simulink model "model2bf"  (R2024b)
settings: Solver=ode4  StartTime=0.0  StopTime=20  FixedStep=2e-3  MaxStep=1e-1  RelTol=1e-3
values from neighbouring files (symbols this model uses):
  Aero = struct    [model2_dim.m]
  brake = struct    [model2_dim.m]
  drivetrain = struct    [model2_dim.m]
  g = 9.81    [model2_dim.m]
  G29 = struct    [model2_dim.m]
  hub_offset = 2.5    [model2_dim.m]
  motor = struct    [model2_dim.m]
  slope_angle = 0    [model2_dim.m]
  suspension = struct    [model2_dim.m]
  tyre = struct    [model2_dim.m]
  vehicle = struct    [model2_dim.m]
  Y = [vehicle.mt * 9.81; 0]    [braking_dyn.m]
undefined symbols (not defined in the file or in its folder): table, wheel, X, Z
libraries: sm_lib x154, nesl_utility x46, simulink x8, slrealtimeG29lib x1, Contact_Forces_Lib x1
(part 5 of 6)

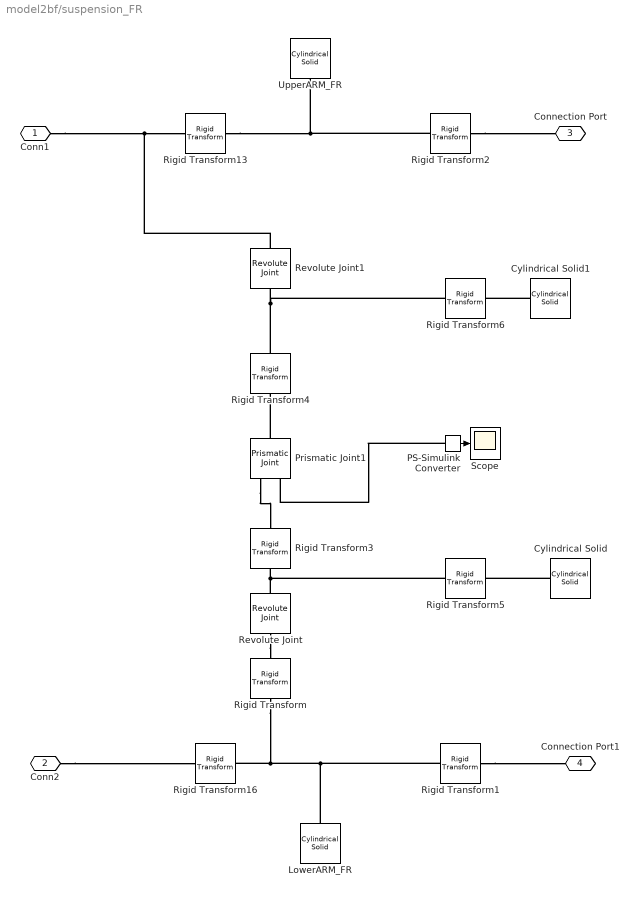
== system model2bf/suspension_FR ==
  Cylindrical Solid : sm_lib/Body Elements/Cylindrical Solid  CylinderRadius=1.5  CylinderRadiusUnits=cm  CylinderLength=15  CylinderLengthUnits=cm  ExportEntireGeometry=off  InertiaType=CalculateFromGeometry  BasedOnType=Density  Density=1000  DensityUnits=kg/m^3  Mass=1  MassUnits=kg  CenterOfMass=[0 0 0]  CenterOfMassUnits=m  MomentsOfInertia=[1 1 1]  MomentsOfInertiaUnits=kg*m^2  ProductsOfInertia=[0 0 0]  ProductsOfInertiaUnits=kg*m^2  GraphicType=FromGeometry  MarkerShape=Sphere  MarkerSize=10  GraphicVisPropType=SimpleVisualProperties  GraphicDiffuseColor=[0 0 1]  GraphicOpacity=1  GraphicSpecularColor=[0.5 0.5 0.5 1.0]  GraphicAmbientColor=[0.15 0.15 0.15 1.0]  GraphicEmissiveColor=[0.0 0.0 0.0 1.0]  GraphicShininess=75  DoExposeReferenceFrame=on  SerializedFrames=<Frames/>
  Cylindrical Solid1 : sm_lib/Body Elements/Cylindrical Solid  CylinderRadius=1  CylinderRadiusUnits=cm  CylinderLength=15  CylinderLengthUnits=cm  ExportEntireGeometry=off  InertiaType=CalculateFromGeometry  BasedOnType=Density  Density=1000  DensityUnits=kg/m^3  Mass=1  MassUnits=kg  CenterOfMass=[0 0 0]  CenterOfMassUnits=m  MomentsOfInertia=[1 1 1]  MomentsOfInertiaUnits=kg*m^2  ProductsOfInertia=[0 0 0]  ProductsOfInertiaUnits=kg*m^2  GraphicType=FromGeometry  MarkerShape=Sphere  MarkerSize=10  GraphicVisPropType=SimpleVisualProperties  GraphicDiffuseColor=[0.07451 0.6235 1]  GraphicOpacity=1  GraphicSpecularColor=[0.5 0.5 0.5 1.0]  GraphicAmbientColor=[0.15 0.15 0.15 1.0]  GraphicEmissiveColor=[0.0 0.0 0.0 1.0]  GraphicShininess=75  DoExposeReferenceFrame=on  SerializedFrames=<Frames/>
  LowerARM_FR : sm_lib/Body Elements/Cylindrical Solid  CylinderRadius=suspension.front.lower.radius  CylinderRadiusUnits=cm  CylinderLength=suspension.front.lower.length  CylinderLengthUnits=cm  ExportEntireGeometry=off  InertiaType=CalculateFromGeometry  BasedOnType=Density  Density=2700  DensityUnits=kg/m^3  Mass=1  MassUnits=kg  CenterOfMass=[0 0 0]  CenterOfMassUnits=m  MomentsOfInertia=[1 1 1]  MomentsOfInertiaUnits=kg*m^2  ProductsOfInertia=[0 0 0]  ProductsOfInertiaUnits=kg*m^2  GraphicType=FromGeometry  MarkerShape=Sphere  MarkerSize=10  GraphicVisPropType=SimpleVisualProperties  GraphicDiffuseColor=[0.5 0.5 0.5]  GraphicOpacity=1  GraphicSpecularColor=[0.5 0.5 0.5 1.0]  GraphicAmbientColor=[0.15 0.15 0.15 1.0]  GraphicEmissiveColor=[0.0 0.0 0.0 1.0]  GraphicShininess=75  DoExposeReferenceFrame=on  SerializedFrames=<Frames/>
  PS-Simulink Converter : nesl_utility/PS-Simulink Converter  PhysicalDomain=network_engine_domain  SubClassName=ps_output  LeftPortType=input  RightPortType=output  PseudoPeriodic=off  Frequencies=[]  VectorFormat=inherit  Unit=inherit  AffineConversion=off
  Prismatic Joint1 : sm_lib/Joints/Prismatic Joint  JointMode=Normal  CompositeWrenchDir=FollowerOnBase  CompositeWrenchFrame=BaseFrame  SenseConstraintForce=off  SenseConstraintTorque=off  SenseTotalForce=off  SenseTotalTorque=off  PositionTargetSpecify=off  PositionTargetPriority=High  PositionTargetValue=0  PositionTargetValueUnits=m  VelocityTargetSpecify=off  VelocityTargetPriority=High  VelocityTargetValue=0  VelocityTargetValueUnits=m/s  EquilibriumPosition=suspension.front.eq  EquilibriumPositionUnits=m  SpringStiffness=suspension.front.stiffness  SpringStiffnessUnits=N/m  DampingCoefficient=suspension.front.damping  DampingCoefficientUnits=N/(m/s)  LowerLimitSpecify=off  LowerLimitBound=-1  LowerLimitBoundUnits=m  LowerLimitStiffness=1e6  LowerLimitStiffnessUnits=N/m  LowerLimitDamping=1e3  LowerLimitDampingUnits=N/(m/s)  LowerLimitTransitionRegionWidth=1e-4  LowerLimitTransitionRegionWidthUnits=m  UpperLimitSpecify=off  UpperLimitBound=1  UpperLimitBoundUnits=m  UpperLimitStiffness=1e6  UpperLimitStiffnessUnits=N/m  UpperLimitDamping=1e3  UpperLimitDampingUnits=N/(m/s)  UpperLimitTransitionRegionWidth=1e-4  UpperLimitTransitionRegionWidthUnits=m  TorqueActuationMode=NoTorque  MotionActuationMode=ComputedMotion  SensePosition=on  SenseVelocity=off  SenseAcceleration=off  SenseTorqueForce=off  SenseLowerLimitTorqueForce=off  SenseUpperLimitTorqueForce=off
  Revolute Joint : sm_lib/Joints/Revolute Joint  JointMode=Normal  CompositeWrenchDir=FollowerOnBase  CompositeWrenchFrame=BaseFrame  SenseConstraintForce=off  SenseConstraintTorque=off  SenseTotalForce=off  SenseTotalTorque=off  PositionTargetSpecify=off  PositionTargetPriority=High  PositionTargetValue=0  PositionTargetValueUnits=deg  VelocityTargetSpecify=off  VelocityTargetPriority=High  VelocityTargetValue=0  VelocityTargetValueUnits=deg/s  EquilibriumPosition=0  EquilibriumPositionUnits=deg  SpringStiffness=0  SpringStiffnessUnits=N*m/deg  DampingCoefficient=0  DampingCoefficientUnits=N*m/(deg/s)  LowerLimitSpecify=off  LowerLimitBound=-90  LowerLimitBoundUnits=deg  LowerLimitStiffness=1e4  LowerLimitStiffnessUnits=N*m/deg  LowerLimitDamping=10  LowerLimitDampingUnits=N*m/(deg/s)  LowerLimitTransitionRegionWidth=0.1  LowerLimitTransitionRegionWidthUnits=deg  UpperLimitSpecify=off  UpperLimitBound=90  UpperLimitBoundUnits=deg  UpperLimitStiffness=1e4  UpperLimitStiffnessUnits=N*m/deg  UpperLimitDamping=10  UpperLimitDampingUnits=N*m/(deg/s)  UpperLimitTransitionRegionWidth=0.1  UpperLimitTransitionRegionWidthUnits=deg  TorqueActuationMode=NoTorque  MotionActuationMode=ComputedMotion  SensePosition=off  SenseVelocity=off  SenseAcceleration=off  SenseTorqueForce=off  SenseLowerLimitTorqueForce=off  SenseUpperLimitTorqueForce=off
  Revolute Joint1 : sm_lib/Joints/Revolute Joint  JointMode=Normal  CompositeWrenchDir=FollowerOnBase  CompositeWrenchFrame=BaseFrame  SenseConstraintForce=off  SenseConstraintTorque=off  SenseTotalForce=off  SenseTotalTorque=off  PositionTargetSpecify=off  PositionTargetPriority=High  PositionTargetValue=0  PositionTargetValueUnits=deg  VelocityTargetSpecify=off  VelocityTargetPriority=High  VelocityTargetValue=0  VelocityTargetValueUnits=deg/s  EquilibriumPosition=0  EquilibriumPositionUnits=deg  SpringStiffness=0  SpringStiffnessUnits=N*m/deg  DampingCoefficient=0  DampingCoefficientUnits=N*m/(deg/s)  LowerLimitSpecify=off  LowerLimitBound=-90  LowerLimitBoundUnits=deg  LowerLimitStiffness=1e4  LowerLimitStiffnessUnits=N*m/deg  LowerLimitDamping=10  LowerLimitDampingUnits=N*m/(deg/s)  LowerLimitTransitionRegionWidth=0.1  LowerLimitTransitionRegionWidthUnits=deg  UpperLimitSpecify=off  UpperLimitBound=90  UpperLimitBoundUnits=deg  UpperLimitStiffness=1e4  UpperLimitStiffnessUnits=N*m/deg  UpperLimitDamping=10  UpperLimitDampingUnits=N*m/(deg/s)  UpperLimitTransitionRegionWidth=0.1  UpperLimitTransitionRegionWidthUnits=deg  TorqueActuationMode=NoTorque  MotionActuationMode=ComputedMotion  SensePosition=off  SenseVelocity=off  SenseAcceleration=off  SenseTorqueForce=off  SenseLowerLimitTorqueForce=off  SenseUpperLimitTorqueForce=off
  Rigid Transform : sm_lib/Frames and Transforms/Rigid Transform  RotationMethod=StandardAxis  FollAlignAxisA=+X  BaseAlignAxisA=+Y  FollAlignAxisB=+Y  BaseAlignAxisB=+Z  RotationStandardAxis=+X  RotationAngle=-90  RotationAngleUnits=deg  RotationArbitraryAxis=[0 0 1]  RotationSequenceAxes=FollowerAxes  RotationSequence=XYX  RotationSequenceAngles=[0 0 0]  RotationSequenceAnglesUnits=deg  RotationMatrix=[1 0 0;0 1 0;0 0 1]  Quaternion=[1 0 0 0]  TranslationMethod=Cartesian  TranslationCartesianOffset=[0 0 -suspension.front.distance_revolute]  TranslationCartesianOffsetUnits=cm  TranslationStandardAxis=+Z  TranslationStandardOffset=0  TranslationStandardOffsetUnits=m  TranslationROffset=0  TranslationROffsetUnits=m  TranslationThetaOffset=0  TranslationThetaOffsetUnits=deg  TranslationZOffset=0  TranslationZOffsetUnits=m
  Rigid Transform1 : sm_lib/Frames and Transforms/Rigid Transform  RotationMethod=RotationSequence  FollAlignAxisA=+X  BaseAlignAxisA=+Y  FollAlignAxisB=+Y  BaseAlignAxisB=+Z  RotationStandardAxis=+X  RotationAngle=90  RotationAngleUnits=deg  RotationArbitraryAxis=[0 0 1]  RotationSequenceAxes=FollowerAxes  RotationSequence=XZX  RotationSequenceAngles=[90 suspension.front.lower.inclination 0]  RotationSequenceAnglesUnits=deg  RotationMatrix=[1 0 0;0 1 0;0 0 1]  Quaternion=[1 0 0 0]  TranslationMethod=Cartesian  TranslationCartesianOffset=[0 0 suspension.front.lower.length/2]  TranslationCartesianOffsetUnits=cm  TranslationStandardAxis=+Z  TranslationStandardOffset=0  TranslationStandardOffsetUnits=m  TranslationROffset=0  TranslationROffsetUnits=m  TranslationThetaOffset=0  TranslationThetaOffsetUnits=deg  TranslationZOffset=0  TranslationZOffsetUnits=m
  Rigid Transform13 : sm_lib/Frames and Transforms/Rigid Transform  RotationMethod=StandardAxis  FollAlignAxisA=+X  BaseAlignAxisA=+Y  FollAlignAxisB=+Y  BaseAlignAxisB=+Z  RotationStandardAxis=+X  RotationAngle=90  RotationAngleUnits=deg  RotationArbitraryAxis=[0 0 1]  RotationSequenceAxes=FollowerAxes  RotationSequence=XYX  RotationSequenceAngles=[0 0 0]  RotationSequenceAnglesUnits=deg  RotationMatrix=[1 0 0;0 1 0;0 0 1]  Quaternion=[1 0 0 0]  TranslationMethod=Cartesian  TranslationCartesianOffset=[0 -suspension.front.upper.length/2 0]  TranslationCartesianOffsetUnits=cm  TranslationStandardAxis=+Z  TranslationStandardOffset=0  TranslationStandardOffsetUnits=m  TranslationROffset=0  TranslationROffsetUnits=m  TranslationThetaOffset=0  TranslationThetaOffsetUnits=deg  TranslationZOffset=0  TranslationZOffsetUnits=m
  Rigid Transform16 : sm_lib/Frames and Transforms/Rigid Transform  RotationMethod=StandardAxis  FollAlignAxisA=+X  BaseAlignAxisA=+Y  FollAlignAxisB=+Y  BaseAlignAxisB=+Z  RotationStandardAxis=+X  RotationAngle=90  RotationAngleUnits=deg  RotationArbitraryAxis=[0 0 1]  RotationSequenceAxes=FollowerAxes  RotationSequence=XYX  RotationSequenceAngles=[0 0 0]  RotationSequenceAnglesUnits=deg  RotationMatrix=[1 0 0;0 1 0;0 0 1]  Quaternion=[1 0 0 0]  TranslationMethod=Cartesian  TranslationCartesianOffset=[0 -suspension.front.lower.length/2 0]  TranslationCartesianOffsetUnits=cm  TranslationStandardAxis=+Z  TranslationStandardOffset=0  TranslationStandardOffsetUnits=m  TranslationROffset=0  TranslationROffsetUnits=m  TranslationThetaOffset=0  TranslationThetaOffsetUnits=deg  TranslationZOffset=0  TranslationZOffsetUnits=m
  Rigid Transform2 : sm_lib/Frames and Transforms/Rigid Transform  RotationMethod=RotationSequence  FollAlignAxisA=+X  BaseAlignAxisA=+Y  FollAlignAxisB=+Y  BaseAlignAxisB=+Z  RotationStandardAxis=+X  RotationAngle=90  RotationAngleUnits=deg  RotationArbitraryAxis=[0 0 1]  RotationSequenceAxes=FollowerAxes  RotationSequence=XZX  RotationSequenceAngles=[90 suspension.front.upper.inclination 0]  RotationSequenceAnglesUnits=deg  RotationMatrix=[1 0 0;0 1 0;0 0 1]  Quaternion=[1 0 0 0]  TranslationMethod=Cartesian  TranslationCartesianOffset=[0 0 suspension.front.upper.length/2]  TranslationCartesianOffsetUnits=cm  TranslationStandardAxis=+Z  TranslationStandardOffset=0  TranslationStandardOffsetUnits=m  TranslationROffset=0  TranslationROffsetUnits=m  TranslationThetaOffset=0  TranslationThetaOffsetUnits=deg  TranslationZOffset=0  TranslationZOffsetUnits=m
  Rigid Transform3 : sm_lib/Frames and Transforms/Rigid Transform  RotationMethod=AlignedAxes  FollAlignAxisA=+Z  BaseAlignAxisA=-X  FollAlignAxisB=+Y  BaseAlignAxisB=+Z  RotationStandardAxis=+Y  RotationAngle=-90  RotationAngleUnits=deg  RotationArbitraryAxis=[0 0 1]  RotationSequenceAxes=FollowerAxes  RotationSequence=XYX  RotationSequenceAngles=[0 0 0]  RotationSequenceAnglesUnits=deg  RotationMatrix=[1 0 0;0 1 0;0 0 1]  Quaternion=[1 0 0 0]  TranslationMethod=None  TranslationCartesianOffset=[0 0 0]  TranslationCartesianOffsetUnits=m  TranslationStandardAxis=+Z  TranslationStandardOffset=0  TranslationStandardOffsetUnits=m  TranslationROffset=0  TranslationROffsetUnits=m  TranslationThetaOffset=0  TranslationThetaOffsetUnits=deg  TranslationZOffset=0  TranslationZOffsetUnits=m
  Rigid Transform4 : sm_lib/Frames and Transforms/Rigid Transform  RotationMethod=StandardAxis  FollAlignAxisA=+X  BaseAlignAxisA=+Y  FollAlignAxisB=+Y  BaseAlignAxisB=+Z  RotationStandardAxis=+X  RotationAngle=90  RotationAngleUnits=deg  RotationArbitraryAxis=[0 0 1]  RotationSequenceAxes=FollowerAxes  RotationSequence=XYX  RotationSequenceAngles=[0 0 0]  RotationSequenceAnglesUnits=deg  RotationMatrix=[1 0 0;0 1 0;0 0 1]  Quaternion=[1 0 0 0]  TranslationMethod=None  TranslationCartesianOffset=[0 0 0]  TranslationCartesianOffsetUnits=m  TranslationStandardAxis=+Z  TranslationStandardOffset=0  TranslationStandardOffsetUnits=m  TranslationROffset=0  TranslationROffsetUnits=m  TranslationThetaOffset=0  TranslationThetaOffsetUnits=deg  TranslationZOffset=0  TranslationZOffsetUnits=m
  Rigid Transform5 : sm_lib/Frames and Transforms/Rigid Transform  RotationMethod=StandardAxis  FollAlignAxisA=+X  BaseAlignAxisA=+Y  FollAlignAxisB=+Y  BaseAlignAxisB=+Z  RotationStandardAxis=+Y  RotationAngle=90  RotationAngleUnits=deg  RotationArbitraryAxis=[0 0 1]  RotationSequenceAxes=FollowerAxes  RotationSequence=XYX  RotationSequenceAngles=[0 0 0]  RotationSequenceAnglesUnits=deg  RotationMatrix=[1 0 0;0 1 0;0 0 1]  Quaternion=[1 0 0 0]  TranslationMethod=Cartesian  TranslationCartesianOffset=[0 0 7.5]  TranslationCartesianOffsetUnits=cm  TranslationStandardAxis=+Z  TranslationStandardOffset=0  TranslationStandardOffsetUnits=m  TranslationROffset=0  TranslationROffsetUnits=m  TranslationThetaOffset=0  TranslationThetaOffsetUnits=deg  TranslationZOffset=0  TranslationZOffsetUnits=m
  Rigid Transform6 : sm_lib/Frames and Transforms/Rigid Transform  RotationMethod=StandardAxis  FollAlignAxisA=+X  BaseAlignAxisA=+Y  FollAlignAxisB=+Y  BaseAlignAxisB=+Z  RotationStandardAxis=+X  RotationAngle=90  RotationAngleUnits=deg  RotationArbitraryAxis=[0 0 1]  RotationSequenceAxes=FollowerAxes  RotationSequence=XYX  RotationSequenceAngles=[0 0 0]  RotationSequenceAnglesUnits=deg  RotationMatrix=[1 0 0;0 1 0;0 0 1]  Quaternion=[1 0 0 0]  TranslationMethod=Cartesian  TranslationCartesianOffset=[0 0 7.5]  TranslationCartesianOffsetUnits=cm  TranslationStandardAxis=+Z  TranslationStandardOffset=0  TranslationStandardOffsetUnits=m  TranslationROffset=0  TranslationROffsetUnits=m  TranslationThetaOffset=0  TranslationThetaOffsetUnits=deg  TranslationZOffset=0  TranslationZOffsetUnits=m
  Scope : Scope
  UpperARM_FR : sm_lib/Body Elements/Cylindrical Solid  CylinderRadius=suspension.front.upper.radius  CylinderRadiusUnits=cm  CylinderLength=suspension.front.upper.length  CylinderLengthUnits=cm  ExportEntireGeometry=off  InertiaType=CalculateFromGeometry  BasedOnType=Density  Density=2700  DensityUnits=kg/m^3  Mass=1  MassUnits=kg  CenterOfMass=[0 0 0]  CenterOfMassUnits=m  MomentsOfInertia=[1 1 1]  MomentsOfInertiaUnits=kg*m^2  ProductsOfInertia=[0 0 0]  ProductsOfInertiaUnits=kg*m^2  GraphicType=FromGeometry  MarkerShape=Sphere  MarkerSize=10  GraphicVisPropType=SimpleVisualProperties  GraphicDiffuseColor=[1 0.4118 0.1608]  GraphicOpacity=1  GraphicSpecularColor=[0.5 0.5 0.5 1.0]  GraphicAmbientColor=[0.15 0.15 0.15 1.0]  GraphicEmissiveColor=[0.0 0.0 0.0 1.0]  GraphicShininess=75  DoExposeReferenceFrame=on  SerializedFrames=<Frames/>
  Conn1 : PMIOPort  Side=Left
  Conn2 : PMIOPort  Port=2  Side=Left
  Connection Port : PMIOPort  Port=3  Side=Right
  Connection Port1 : PMIOPort  Port=4  Side=Right
  wires:
  PS-Simulink Converter/1 -> Scope/1
  connections:
  Conn1/RConn1 -- Revolute Joint1/LConn1 -- Rigid Transform13/LConn1
  Conn2/RConn1 -- Rigid Transform16/LConn1
  LowerARM_FR/RConn1 -- Rigid Transform16/RConn1 -- Rigid Transform/LConn1 -- Rigid Transform1/LConn1
  Rigid Transform13/RConn1 -- Rigid Transform2/LConn1 -- UpperARM_FR/RConn1
  Rigid Transform1/RConn1 -- Connection Port1/RConn1
  Rigid Transform2/RConn1 -- Connection Port/RConn1
  Revolute Joint/LConn1 -- Rigid Transform5/RConn1 -- Rigid Transform3/LConn1
  Rigid Transform4/LConn1 -- Rigid Transform6/RConn1 -- Revolute Joint1/RConn1
  Cylindrical Solid1/RConn1 -- Rigid Transform6/LConn1
  Prismatic Joint1/LConn1 -- Rigid Transform4/RConn1
  Revolute Joint/RConn1 -- Rigid Transform/RConn1
  Cylindrical Solid/RConn1 -- Rigid Transform5/LConn1
  Prismatic Joint1/RConn1 -- Rigid Transform3/RConn1
  PS-Simulink Converter/LConn1 -- Prismatic Joint1/RConn2

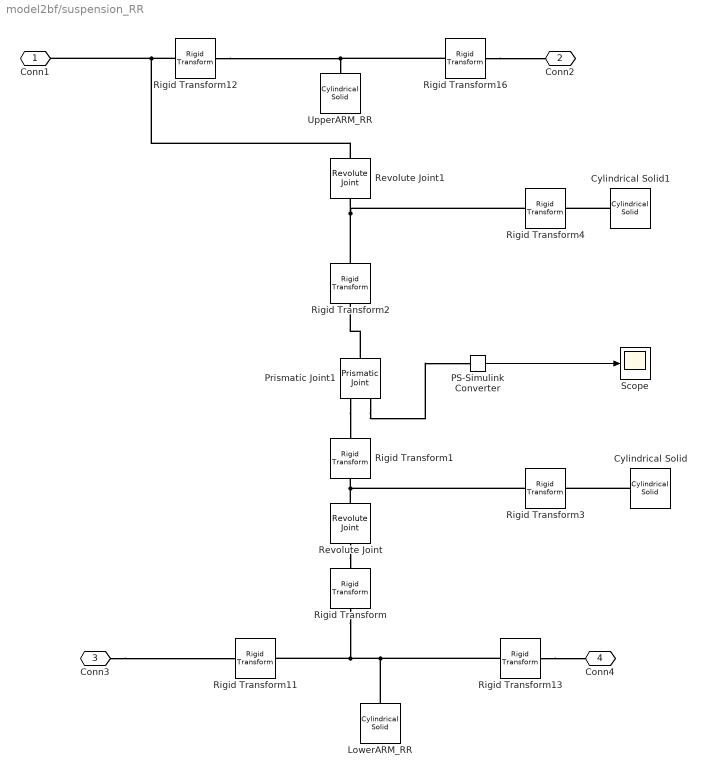
== system model2bf/suspension_RR ==
  Cylindrical Solid : sm_lib/Body Elements/Cylindrical Solid  CylinderRadius=1.5  CylinderRadiusUnits=cm  CylinderLength=15  CylinderLengthUnits=cm  ExportEntireGeometry=off  InertiaType=CalculateFromGeometry  BasedOnType=Density  Density=1000  DensityUnits=kg/m^3  Mass=1  MassUnits=kg  CenterOfMass=[0 0 0]  CenterOfMassUnits=m  MomentsOfInertia=[1 1 1]  MomentsOfInertiaUnits=kg*m^2  ProductsOfInertia=[0 0 0]  ProductsOfInertiaUnits=kg*m^2  GraphicType=FromGeometry  MarkerShape=Sphere  MarkerSize=10  GraphicVisPropType=SimpleVisualProperties  GraphicDiffuseColor=[0 0 1]  GraphicOpacity=1  GraphicSpecularColor=[0.5 0.5 0.5 1.0]  GraphicAmbientColor=[0.15 0.15 0.15 1.0]  GraphicEmissiveColor=[0.0 0.0 0.0 1.0]  GraphicShininess=75  DoExposeReferenceFrame=on  SerializedFrames=<Frames/>
  Cylindrical Solid1 : sm_lib/Body Elements/Cylindrical Solid  CylinderRadius=1  CylinderRadiusUnits=cm  CylinderLength=15  CylinderLengthUnits=cm  ExportEntireGeometry=off  InertiaType=CalculateFromGeometry  BasedOnType=Density  Density=1000  DensityUnits=kg/m^3  Mass=1  MassUnits=kg  CenterOfMass=[0 0 0]  CenterOfMassUnits=m  MomentsOfInertia=[1 1 1]  MomentsOfInertiaUnits=kg*m^2  ProductsOfInertia=[0 0 0]  ProductsOfInertiaUnits=kg*m^2  GraphicType=FromGeometry  MarkerShape=Sphere  MarkerSize=10  GraphicVisPropType=SimpleVisualProperties  GraphicDiffuseColor=[0.07451 0.6235 1]  GraphicOpacity=1  GraphicSpecularColor=[0.5 0.5 0.5 1.0]  GraphicAmbientColor=[0.15 0.15 0.15 1.0]  GraphicEmissiveColor=[0.0 0.0 0.0 1.0]  GraphicShininess=75  DoExposeReferenceFrame=on  SerializedFrames=<Frames/>
  LowerARM_RR : sm_lib/Body Elements/Cylindrical Solid  CylinderRadius=suspension.rear.lower.radius  CylinderRadiusUnits=cm  CylinderLength=suspension.rear.lower.length  CylinderLengthUnits=cm  ExportEntireGeometry=off  InertiaType=CalculateFromGeometry  BasedOnType=Density  Density=2700  DensityUnits=kg/m^3  Mass=1  MassUnits=kg  CenterOfMass=[0 0 0]  CenterOfMassUnits=m  MomentsOfInertia=[1 1 1]  MomentsOfInertiaUnits=kg*m^2  ProductsOfInertia=[0 0 0]  ProductsOfInertiaUnits=kg*m^2  GraphicType=FromGeometry  MarkerShape=Sphere  MarkerSize=10  GraphicVisPropType=SimpleVisualProperties  GraphicDiffuseColor=[0.5 0.5 0.5]  GraphicOpacity=1  GraphicSpecularColor=[0.5 0.5 0.5 1.0]  GraphicAmbientColor=[0.15 0.15 0.15 1.0]  GraphicEmissiveColor=[0.0 0.0 0.0 1.0]  GraphicShininess=75  DoExposeReferenceFrame=on  SerializedFrames=<Frames/>
  PS-Simulink Converter : nesl_utility/PS-Simulink Converter  PhysicalDomain=network_engine_domain  SubClassName=ps_output  LeftPortType=input  RightPortType=output  PseudoPeriodic=off  Frequencies=[]  VectorFormat=inherit  Unit=inherit  AffineConversion=off
  Prismatic Joint1 : sm_lib/Joints/Prismatic Joint  JointMode=Normal  CompositeWrenchDir=FollowerOnBase  CompositeWrenchFrame=BaseFrame  SenseConstraintForce=off  SenseConstraintTorque=off  SenseTotalForce=off  SenseTotalTorque=off  PositionTargetSpecify=off  PositionTargetPriority=High  PositionTargetValue=0  PositionTargetValueUnits=m  VelocityTargetSpecify=off  VelocityTargetPriority=High  VelocityTargetValue=0  VelocityTargetValueUnits=m/s  EquilibriumPosition=suspension.rear.eq  EquilibriumPositionUnits=m  SpringStiffness=suspension.rear.stiffness  SpringStiffnessUnits=N/m  DampingCoefficient=suspension.rear.damping  DampingCoefficientUnits=N/(m/s)  LowerLimitSpecify=off  LowerLimitBound=-1  LowerLimitBoundUnits=m  LowerLimitStiffness=1e6  LowerLimitStiffnessUnits=N/m  LowerLimitDamping=1e3  LowerLimitDampingUnits=N/(m/s)  LowerLimitTransitionRegionWidth=1e-4  LowerLimitTransitionRegionWidthUnits=m  UpperLimitSpecify=off  UpperLimitBound=1  UpperLimitBoundUnits=m  UpperLimitStiffness=1e6  UpperLimitStiffnessUnits=N/m  UpperLimitDamping=1e3  UpperLimitDampingUnits=N/(m/s)  UpperLimitTransitionRegionWidth=1e-4  UpperLimitTransitionRegionWidthUnits=m  TorqueActuationMode=NoTorque  MotionActuationMode=ComputedMotion  SensePosition=on  SenseVelocity=off  SenseAcceleration=off  SenseTorqueForce=off  SenseLowerLimitTorqueForce=off  SenseUpperLimitTorqueForce=off
  Revolute Joint : sm_lib/Joints/Revolute Joint  JointMode=Normal  CompositeWrenchDir=FollowerOnBase  CompositeWrenchFrame=BaseFrame  SenseConstraintForce=off  SenseConstraintTorque=off  SenseTotalForce=off  SenseTotalTorque=off  PositionTargetSpecify=off  PositionTargetPriority=High  PositionTargetValue=0  PositionTargetValueUnits=deg  VelocityTargetSpecify=off  VelocityTargetPriority=High  VelocityTargetValue=0  VelocityTargetValueUnits=deg/s  EquilibriumPosition=0  EquilibriumPositionUnits=deg  SpringStiffness=0  SpringStiffnessUnits=N*m/deg  DampingCoefficient=0  DampingCoefficientUnits=N*m/(deg/s)  LowerLimitSpecify=off  LowerLimitBound=-90  LowerLimitBoundUnits=deg  LowerLimitStiffness=1e4  LowerLimitStiffnessUnits=N*m/deg  LowerLimitDamping=10  LowerLimitDampingUnits=N*m/(deg/s)  LowerLimitTransitionRegionWidth=0.1  LowerLimitTransitionRegionWidthUnits=deg  UpperLimitSpecify=off  UpperLimitBound=90  UpperLimitBoundUnits=deg  UpperLimitStiffness=1e4  UpperLimitStiffnessUnits=N*m/deg  UpperLimitDamping=10  UpperLimitDampingUnits=N*m/(deg/s)  UpperLimitTransitionRegionWidth=0.1  UpperLimitTransitionRegionWidthUnits=deg  TorqueActuationMode=NoTorque  MotionActuationMode=ComputedMotion  SensePosition=off  SenseVelocity=off  SenseAcceleration=off  SenseTorqueForce=off  SenseLowerLimitTorqueForce=off  SenseUpperLimitTorqueForce=off
  Revolute Joint1 : sm_lib/Joints/Revolute Joint  JointMode=Normal  CompositeWrenchDir=FollowerOnBase  CompositeWrenchFrame=BaseFrame  SenseConstraintForce=off  SenseConstraintTorque=off  SenseTotalForce=off  SenseTotalTorque=off  PositionTargetSpecify=off  PositionTargetPriority=High  PositionTargetValue=0  PositionTargetValueUnits=deg  VelocityTargetSpecify=off  VelocityTargetPriority=High  VelocityTargetValue=0  VelocityTargetValueUnits=deg/s  EquilibriumPosition=0  EquilibriumPositionUnits=deg  SpringStiffness=0  SpringStiffnessUnits=N*m/deg  DampingCoefficient=0  DampingCoefficientUnits=N*m/(deg/s)  LowerLimitSpecify=off  LowerLimitBound=-90  LowerLimitBoundUnits=deg  LowerLimitStiffness=1e4  LowerLimitStiffnessUnits=N*m/deg  LowerLimitDamping=10  LowerLimitDampingUnits=N*m/(deg/s)  LowerLimitTransitionRegionWidth=0.1  LowerLimitTransitionRegionWidthUnits=deg  UpperLimitSpecify=off  UpperLimitBound=90  UpperLimitBoundUnits=deg  UpperLimitStiffness=1e4  UpperLimitStiffnessUnits=N*m/deg  UpperLimitDamping=10  UpperLimitDampingUnits=N*m/(deg/s)  UpperLimitTransitionRegionWidth=0.1  UpperLimitTransitionRegionWidthUnits=deg  TorqueActuationMode=NoTorque  MotionActuationMode=ComputedMotion  SensePosition=off  SenseVelocity=off  SenseAcceleration=off  SenseTorqueForce=off  SenseLowerLimitTorqueForce=off  SenseUpperLimitTorqueForce=off
  Rigid Transform : sm_lib/Frames and Transforms/Rigid Transform  RotationMethod=StandardAxis  FollAlignAxisA=+X  BaseAlignAxisA=+Y  FollAlignAxisB=+Y  BaseAlignAxisB=+Z  RotationStandardAxis=+X  RotationAngle=-90  RotationAngleUnits=deg  RotationArbitraryAxis=[0 0 1]  RotationSequenceAxes=FollowerAxes  RotationSequence=XYX  RotationSequenceAngles=[0 0 0]  RotationSequenceAnglesUnits=deg  RotationMatrix=[1 0 0;0 1 0;0 0 1]  Quaternion=[1 0 0 0]  TranslationMethod=Cartesian  TranslationCartesianOffset=[0 0 -suspension.rear.distance_revolute]  TranslationCartesianOffsetUnits=cm  TranslationStandardAxis=+Z  TranslationStandardOffset=0  TranslationStandardOffsetUnits=m  TranslationROffset=0  TranslationROffsetUnits=m  TranslationThetaOffset=0  TranslationThetaOffsetUnits=deg  TranslationZOffset=0  TranslationZOffsetUnits=m
  Rigid Transform1 : sm_lib/Frames and Transforms/Rigid Transform  RotationMethod=AlignedAxes  FollAlignAxisA=+Z  BaseAlignAxisA=-X  FollAlignAxisB=+Y  BaseAlignAxisB=+Z  RotationStandardAxis=+Y  RotationAngle=-90  RotationAngleUnits=deg  RotationArbitraryAxis=[0 0 1]  RotationSequenceAxes=FollowerAxes  RotationSequence=XYX  RotationSequenceAngles=[0 0 0]  RotationSequenceAnglesUnits=deg  RotationMatrix=[1 0 0;0 1 0;0 0 1]  Quaternion=[1 0 0 0]  TranslationMethod=None  TranslationCartesianOffset=[0 0 0]  TranslationCartesianOffsetUnits=m  TranslationStandardAxis=+Z  TranslationStandardOffset=0  TranslationStandardOffsetUnits=m  TranslationROffset=0  TranslationROffsetUnits=m  TranslationThetaOffset=0  TranslationThetaOffsetUnits=deg  TranslationZOffset=0  TranslationZOffsetUnits=m
  Rigid Transform11 : sm_lib/Frames and Transforms/Rigid Transform  RotationMethod=StandardAxis  FollAlignAxisA=+X  BaseAlignAxisA=+Y  FollAlignAxisB=+Y  BaseAlignAxisB=+Z  RotationStandardAxis=+X  RotationAngle=90  RotationAngleUnits=deg  RotationArbitraryAxis=[0 0 1]  RotationSequenceAxes=FollowerAxes  RotationSequence=XYX  RotationSequenceAngles=[0 0 0]  RotationSequenceAnglesUnits=deg  RotationMatrix=[1 0 0;0 1 0;0 0 1]  Quaternion=[1 0 0 0]  TranslationMethod=Cartesian  TranslationCartesianOffset=[0 -suspension.rear.lower.length/2 0]  TranslationCartesianOffsetUnits=cm  TranslationStandardAxis=+Z  TranslationStandardOffset=0  TranslationStandardOffsetUnits=m  TranslationROffset=0  TranslationROffsetUnits=m  TranslationThetaOffset=0  TranslationThetaOffsetUnits=deg  TranslationZOffset=0  TranslationZOffsetUnits=m
  Rigid Transform12 : sm_lib/Frames and Transforms/Rigid Transform  RotationMethod=StandardAxis  FollAlignAxisA=+X  BaseAlignAxisA=+Y  FollAlignAxisB=+Y  BaseAlignAxisB=+Z  RotationStandardAxis=+X  RotationAngle=90  RotationAngleUnits=deg  RotationArbitraryAxis=[0 0 1]  RotationSequenceAxes=FollowerAxes  RotationSequence=XYX  RotationSequenceAngles=[0 0 0]  RotationSequenceAnglesUnits=deg  RotationMatrix=[1 0 0;0 1 0;0 0 1]  Quaternion=[1 0 0 0]  TranslationMethod=Cartesian  TranslationCartesianOffset=[0 -suspension.rear.upper.length/2 0]  TranslationCartesianOffsetUnits=cm  TranslationStandardAxis=+Z  TranslationStandardOffset=0  TranslationStandardOffsetUnits=m  TranslationROffset=0  TranslationROffsetUnits=m  TranslationThetaOffset=0  TranslationThetaOffsetUnits=deg  TranslationZOffset=0  TranslationZOffsetUnits=m
  Rigid Transform13 : sm_lib/Frames and Transforms/Rigid Transform  RotationMethod=RotationSequence  FollAlignAxisA=+X  BaseAlignAxisA=+Y  FollAlignAxisB=+Y  BaseAlignAxisB=+Z  RotationStandardAxis=+X  RotationAngle=90  RotationAngleUnits=deg  RotationArbitraryAxis=[0 0 1]  RotationSequenceAxes=FollowerAxes  RotationSequence=XZX  RotationSequenceAngles=[90 suspension.rear.lower.inclination 0]  RotationSequenceAnglesUnits=deg  RotationMatrix=[1 0 0;0 1 0;0 0 1]  Quaternion=[1 0 0 0]  TranslationMethod=Cartesian  TranslationCartesianOffset=[0 0 suspension.rear.lower.length/2]  TranslationCartesianOffsetUnits=cm  TranslationStandardAxis=+Z  TranslationStandardOffset=0  TranslationStandardOffsetUnits=m  TranslationROffset=0  TranslationROffsetUnits=m  TranslationThetaOffset=0  TranslationThetaOffsetUnits=deg  TranslationZOffset=0  TranslationZOffsetUnits=m
  Rigid Transform16 : sm_lib/Frames and Transforms/Rigid Transform  RotationMethod=RotationSequence  FollAlignAxisA=+X  BaseAlignAxisA=+Y  FollAlignAxisB=+Y  BaseAlignAxisB=+Z  RotationStandardAxis=+X  RotationAngle=90  RotationAngleUnits=deg  RotationArbitraryAxis=[0 0 1]  RotationSequenceAxes=FollowerAxes  RotationSequence=XZX  RotationSequenceAngles=[90 suspension.rear.upper.inclination 0]  RotationSequenceAnglesUnits=deg  RotationMatrix=[1 0 0;0 1 0;0 0 1]  Quaternion=[1 0 0 0]  TranslationMethod=Cartesian  TranslationCartesianOffset=[0 0 suspension.rear.upper.length/2]  TranslationCartesianOffsetUnits=cm  TranslationStandardAxis=+Z  TranslationStandardOffset=0  TranslationStandardOffsetUnits=m  TranslationROffset=0  TranslationROffsetUnits=m  TranslationThetaOffset=0  TranslationThetaOffsetUnits=deg  TranslationZOffset=0  TranslationZOffsetUnits=m
  Rigid Transform2 : sm_lib/Frames and Transforms/Rigid Transform  RotationMethod=StandardAxis  FollAlignAxisA=+X  BaseAlignAxisA=+Y  FollAlignAxisB=+Y  BaseAlignAxisB=+Z  RotationStandardAxis=+X  RotationAngle=90  RotationAngleUnits=deg  RotationArbitraryAxis=[0 0 1]  RotationSequenceAxes=FollowerAxes  RotationSequence=XYX  RotationSequenceAngles=[0 0 0]  RotationSequenceAnglesUnits=deg  RotationMatrix=[1 0 0;0 1 0;0 0 1]  Quaternion=[1 0 0 0]  TranslationMethod=None  TranslationCartesianOffset=[0 0 0]  TranslationCartesianOffsetUnits=m  TranslationStandardAxis=+Z  TranslationStandardOffset=0  TranslationStandardOffsetUnits=m  TranslationROffset=0  TranslationROffsetUnits=m  TranslationThetaOffset=0  TranslationThetaOffsetUnits=deg  TranslationZOffset=0  TranslationZOffsetUnits=m
  Rigid Transform3 : sm_lib/Frames and Transforms/Rigid Transform  RotationMethod=StandardAxis  FollAlignAxisA=+X  BaseAlignAxisA=+Y  FollAlignAxisB=+Y  BaseAlignAxisB=+Z  RotationStandardAxis=+Y  RotationAngle=90  RotationAngleUnits=deg  RotationArbitraryAxis=[0 0 1]  RotationSequenceAxes=FollowerAxes  RotationSequence=XYX  RotationSequenceAngles=[0 0 0]  RotationSequenceAnglesUnits=deg  RotationMatrix=[1 0 0;0 1 0;0 0 1]  Quaternion=[1 0 0 0]  TranslationMethod=Cartesian  TranslationCartesianOffset=[0 0 7.5]  TranslationCartesianOffsetUnits=cm  TranslationStandardAxis=+Z  TranslationStandardOffset=0  TranslationStandardOffsetUnits=m  TranslationROffset=0  TranslationROffsetUnits=m  TranslationThetaOffset=0  TranslationThetaOffsetUnits=deg  TranslationZOffset=0  TranslationZOffsetUnits=m
  Rigid Transform4 : sm_lib/Frames and Transforms/Rigid Transform  RotationMethod=StandardAxis  FollAlignAxisA=+X  BaseAlignAxisA=+Y  FollAlignAxisB=+Y  BaseAlignAxisB=+Z  RotationStandardAxis=+X  RotationAngle=90  RotationAngleUnits=deg  RotationArbitraryAxis=[0 0 1]  RotationSequenceAxes=FollowerAxes  RotationSequence=XYX  RotationSequenceAngles=[0 0 0]  RotationSequenceAnglesUnits=deg  RotationMatrix=[1 0 0;0 1 0;0 0 1]  Quaternion=[1 0 0 0]  TranslationMethod=Cartesian  TranslationCartesianOffset=[0 0 7.5]  TranslationCartesianOffsetUnits=cm  TranslationStandardAxis=+Z  TranslationStandardOffset=0  TranslationStandardOffsetUnits=m  TranslationROffset=0  TranslationROffsetUnits=m  TranslationThetaOffset=0  TranslationThetaOffsetUnits=deg  TranslationZOffset=0  TranslationZOffsetUnits=m
  Scope : Scope
  UpperARM_RR : sm_lib/Body Elements/Cylindrical Solid  CylinderRadius=suspension.rear.upper.radius  CylinderRadiusUnits=cm  CylinderLength=suspension.rear.upper.length  CylinderLengthUnits=cm  ExportEntireGeometry=off  InertiaType=CalculateFromGeometry  BasedOnType=Density  Density=2700  DensityUnits=kg/m^3  Mass=1  MassUnits=kg  CenterOfMass=[0 0 0]  CenterOfMassUnits=m  MomentsOfInertia=[1 1 1]  MomentsOfInertiaUnits=kg*m^2  ProductsOfInertia=[0 0 0]  ProductsOfInertiaUnits=kg*m^2  GraphicType=FromGeometry  MarkerShape=Sphere  MarkerSize=10  GraphicVisPropType=SimpleVisualProperties  GraphicDiffuseColor=[1 0.4118 0.1608]  GraphicOpacity=1  GraphicSpecularColor=[0.5 0.5 0.5 1.0]  GraphicAmbientColor=[0.15 0.15 0.15 1.0]  GraphicEmissiveColor=[0.0 0.0 0.0 1.0]  GraphicShininess=75  DoExposeReferenceFrame=on  SerializedFrames=<Frames/>
  Conn1 : PMIOPort  Side=Left
  Conn2 : PMIOPort  Port=2  Side=Right
  Conn3 : PMIOPort  Port=3  Side=Left
  Conn4 : PMIOPort  Port=4  Side=Right
  wires:
  PS-Simulink Converter/1 -> Scope/1
  connections:
  Rigid Transform13/RConn1 -- Conn4/RConn1
  Rigid Transform16/RConn1 -- Conn2/RConn1
  LowerARM_RR/RConn1 -- Rigid Transform13/LConn1 -- Rigid Transform/LConn1 -- Rigid Transform11/RConn1
  Rigid Transform12/RConn1 -- Rigid Transform16/LConn1 -- UpperARM_RR/RConn1
  Rigid Transform12/LConn1 -- Conn1/RConn1 -- Revolute Joint1/LConn1
  Conn3/RConn1 -- Rigid Transform11/LConn1
  Revolute Joint/RConn1 -- Rigid Transform/RConn1
  Revolute Joint/LConn1 -- Rigid Transform3/RConn1 -- Rigid Transform1/LConn1
  Rigid Transform2/LConn1 -- Rigid Transform4/RConn1 -- Revolute Joint1/RConn1
  Prismatic Joint1/LConn1 -- Rigid Transform2/RConn1
  Cylindrical Solid/RConn1 -- Rigid Transform3/LConn1
  Cylindrical Solid1/RConn1 -- Rigid Transform4/LConn1
  Prismatic Joint1/RConn1 -- Rigid Transform1/RConn1
  Prismatic Joint1/RConn2 -- PS-Simulink Converter/LConn1

== system model2bf/Chassis/Aero Forces ==
  u : Inport
  Constant : Constant
  Constant1 : Constant  Value=0
  Gain : Gain  Gain=[-Aero.Drag_reduced, 0, Aero.Lift_reduced]
  MATLAB Function : MATLAB Function  TreatAsAtomicUnit=on
  Product : Product
  Switch : Switch  Criteria=u2 > Threshold  SaturateOnIntegerOverflow=off  InputSameDT=off
  Out1 : Outport
  wires:
  MATLAB Function/1(y) -> Switch/2, Product/2
  Constant1/1 -> Switch/3
  Gain/1 -> Out1/1
  Constant/1 -> Switch/1
  Switch/1 -> Product/1
  Product/1 -> Gain/1
  u/1 -> MATLAB Function/1(u)

== system model2bf/Driveline/Acceleration calculation ==
  wheel force : Inport
  Abs : Abs  SaturateOnIntegerOverflow=off
  From : From  Commented=on  GotoTag=Fy_RL  TagVisibility=global
  From1 : From  Commented=on  GotoTag=Fy_RR  TagVisibility=global
  Gain : Gain  Commented=on  Gain=motor.efficiency*motor.gearratio/(tyre.radius/100)
  Gain1 : Gain  Gain=1/((wheel.ir1+wheel.ir2+drivetrain.i_tot*motor.gearratio^2)/((tyre.radius/100)*(tyre.dynamic_radius/100))+vehicle.totalmass)
  MATLAB Function : MATLAB Function  Commented=on  TreatAsAtomicUnit=on
  Min : MinMax  Commented=on  Inputs=2
  Minus : Sum  Inputs=+---
  Rolling coefficient term : Constant  Value=tyre.Cr*vehicle.totalmass*g*cosd(slope_angle)
  Scope : Scope
  Scope1 : Scope
  Slope term : Constant  Value=vehicle.totalmass*g*sind(slope_angle)
  mu_a : Gain  Commented=on  Gain=vehicle.mu_a
  mu_g : Gain  Commented=on  Gain=vehicle.mu_g
  Acceleration : Outport
  wires:
  Rolling coefficient term/1 -> Minus/3
  Slope term/1 -> Minus/4
  Minus/1 -> Gain1/1
  Gain1/1 -> Scope1/1, Acceleration/1
  Min/1 -> mu_g/1, mu_a/1
  mu_a/1 -> MATLAB Function/1(maxforce)
  mu_g/1 -> MATLAB Function/2(limitforce)
  Gain/1 -> MATLAB Function/3(wheelforce)
  wheel force/1 -> Scope/1, Minus/1
  From/1 -> Min/1
  From1/1 -> Min/2
  Abs/1 -> Minus/2
  [F_D] -> Abs/1

== system model2bf/Driveline/Subsystem2 ==
  v (m/s) : Inport
  Braking (%) : Inport  Port=2
  Because we cannot use regen braking at low speed : Switch  Criteria=u2 > Threshold  Threshold=2  SaturateOnIntegerOverflow=off  InputSameDT=off
  Constant : Constant  Value=0
  Gain : Gain  Gain=1 - brake.brakefraction
  Gain1 : Gain  Gain=brake.brakefraction
  Gain2 : Gain  Gain=1/motor.gearratio
  Gain3 : Gain  Gain=brake.pedalratio
  Gain4 : Gain  Gain=1/brake.mastercylinderA
  Gain5 : Gain  Gain=brake.pistonN*brake.pistonA
  Gain6 : Gain  Gain=2*brake.effectiveradius*brake.padfriction
  Gain7 : Gain  Gain=brake.Ffoot_max
  Saturation : Saturate  UpperLimit=0  LowerLimit=-500
  Switch : Switch  Criteria=u2 > Threshold  Threshold=2  SaturateOnIntegerOverflow=off  InputSameDT=off
  FrictionBrake_Tr : Outport
  RegenBrake_Tr : Outport  Port=2
  wires:
  Gain1/1 -> Gain2/1  "RegenBrakeWheel_Tr"
  v (m/s)/1 -> Because we cannot use regen braking at low speed/2, Switch/2
  Constant/1 -> Because we cannot use regen braking at low speed/3
  Switch/1 -> FrictionBrake_Tr/1  "FrictionBrake_Tr"
  Saturation/1 -> RegenBrake_Tr/1  "RegenBrakeTrq"
  Because we cannot use regen braking at low speed/1 -> Saturation/1
  Gain/1 -> Switch/1  "FrictionBrake_Tr"
  Gain6/1 -> Switch/3, Gain1/1, Gain/1  "Total_brake_Tr"
  Gain5/1 -> Gain6/1  "F_clamp"
  Gain4/1 -> Gain5/1  "P_line"
  Gain3/1 -> Gain4/1  "F_pedal"
  Braking (%)/1 -> Gain7/1
  Gain7/1 -> Gain3/1  "F_foot"
  Gain2/1 -> Because we cannot use regen braking at low speed/1  "RegenBrakeMotor_Tr"

== system model2bf/Driveline/Subsystem3 ==
  Motor torque (Nm) : Inport
  Regen Torque : Inport  Port=2
  Throttle (%) : Inport  Port=3
  Add : Sum
  Subsystem : Subsystem
  Torque limit : Subsystem
  MotorTrqOut (Nm) : Outport
  wires:
  Regen Torque/1 -> Subsystem/1(Regen_demand)
  Torque limit/1(Regen_trq_limit) -> Subsystem/2(Regen_Limit)
  Subsystem/1(Regen_Trq) -> Add/1
  Throttle (%)/1 -> Torque limit/1(Throttle (%))
  Motor torque (Nm)/1 -> Torque limit/2(Motor torque (Nm))
  Torque limit/2(Trq_Dmd) -> Add/2
  Add/1 -> MotorTrqOut (Nm)/1  "mech. torque"

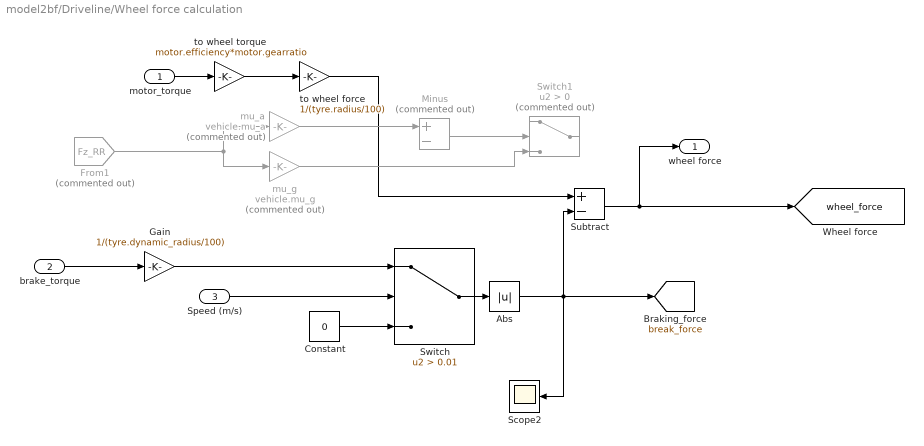
== system model2bf/Driveline/Wheel force calculation ==
  motor_torque : Inport
  brake_torque : Inport  Port=2
  Speed (m/s) : Inport  Port=3
  Abs : Abs  SaturateOnIntegerOverflow=off
  Constant : Constant  Value=0
  From1 : From  Commented=on  GotoTag=Fz_RR  TagVisibility=global
  Gain : Gain  Gain=1/(tyre.dynamic_radius/100)
  Minus : Sum  Commented=on  Inputs=+-
  Scope2 : Scope
  Subtract : Sum  Inputs=+-
  Switch : Switch  Criteria=u2 > Threshold  Threshold=0.01  SaturateOnIntegerOverflow=off  InputSameDT=off
  Switch1 : Switch  Commented=on  Criteria=u2 > Threshold  SaturateOnIntegerOverflow=off  InputSameDT=off
  mu_a : Gain  Commented=on  Gain=vehicle.mu_a
  mu_g : Gain  Commented=on  Gain=vehicle.mu_g
  to wheel force : Gain  Gain=1/(tyre.radius/100)
  to wheel torque : Gain  Gain=motor.efficiency*motor.gearratio
  wheel force : Outport
  tag scope: break_force=global, wheel_force=global
  wires:
  motor_torque/1 -> to wheel torque/1
  to wheel torque/1 -> to wheel force/1
  brake_torque/1 -> Gain/1
  Gain/1 -> Switch/1
  Speed (m/s)/1 -> Switch/2
  Constant/1 -> Switch/3
  Switch/1 -> Abs/1
  to wheel force/1 -> Subtract/1
  Subtract/1 -> wheel force/1, [wheel_force]
  Abs/1 -> Scope2/1, Subtract/2, [break_force]
  From1/1 -> mu_g/1, mu_a/1
  mu_g/1 -> Switch1/3
  mu_a/1 -> Minus/1
  Minus/1 -> Switch1/2

== system model2bf/Tyre FR/Magic formula subsystem ==
  note: SIgn of the steering input
  note: positive force = to the left
  Fz : Inport
  Steering input : Inport  Port=2
  Tyre data : Inport  Port=3
  Bus Selector : BusSelector  OutputSignals=velocity_FR,rotation_FR,inclination_FR
  Constant : Constant  Value=0
  MATLAB Function : MATLAB Function  TreatAsAtomicUnit=on
  Magic formula : MATLAB Function  TreatAsAtomicUnit=on
  Scope : Scope
  Scope1 : Scope
  Sum : Sum
  Switch : Switch  Criteria=u2 > Threshold  Threshold=0.5  SaturateOnIntegerOverflow=off  InputSameDT=off
  norm : MATLAB Function  TreatAsAtomicUnit=on
  Force : Outport
  wires:
  Fz/1 -> Magic formula/1(Fz)
  Switch/1 -> Force/1
  norm/1(y) -> Switch/2
  Magic formula/1(Fy) -> Scope/1, Switch/1
  Constant/1 -> Switch/3
  Tyre data/1 -> Bus Selector/1
  Steering input/1 -> Sum/1
  MATLAB Function/1(theta) -> Scope1/1, Sum/2  "slip angle"
  Sum/1 -> Magic formula/2(SA)  "Effective slip angle_FR"
  Bus Selector/1 -> [Speed], MATLAB Function/1(u)  "<velocity_FR>"
  [Speed] -> norm/1(u)
  Bus Selector/2 -> MATLAB Function/2(r)  "<rotation_FR>"
  Bus Selector/3 -> Magic formula/3(Camber)  "<inclination_FR>"

== system model2bf/Tyre_FL/Magic formula subsystem ==
  note: reflection
      | : positive slip = tyre turned to the left = force to the left
  note: SIgn of the steering input
  note: positive force = to the left
  Fz : Inport
  Steering input : Inport  Port=2
  Tyre data : Inport  Port=3
  Bus Selector : BusSelector  OutputSignals=velocity_FL,rotation_FL,inclination_FL
  Constant : Constant  Value=0
  MATLAB Function : MATLAB Function  TreatAsAtomicUnit=on
  Magic formula : MATLAB Function  TreatAsAtomicUnit=on
  Scope : Scope
  Scope1 : Scope
  Sum : Sum
  Switch : Switch  Criteria=u2 > Threshold  Threshold=0.5  SaturateOnIntegerOverflow=off  InputSameDT=off
  norm : MATLAB Function  TreatAsAtomicUnit=on
  Force : Outport
  wires:
  Fz/1 -> Magic formula/1(Fz)
  Switch/1 -> Force/1
  norm/1(y) -> Switch/2
  Magic formula/1(Fy) -> Scope/1, Switch/1
  Constant/1 -> Switch/3
  Tyre data/1 -> Bus Selector/1
  Steering input/1 -> Sum/1
  MATLAB Function/1(theta) -> Sum/2, Scope1/1  "slip angle"
  Sum/1 -> Magic formula/2(SA)  "Effective slip angle_FL"
  Bus Selector/1 -> MATLAB Function/1(u), [Speed]  "<velocity_FL>"
  [Speed] -> norm/1(u)
  Bus Selector/2 -> MATLAB Function/2(r)  "<rotation_FL>"
  Bus Selector/3 -> Magic formula/3(Camber)  "<inclination_FL>"

== system model2bf/Tyre_RL/Magic formula subsystem ==
  note: positive force = to the left
  Fz : Inport
  Tyre data : Inport  Port=2
  Bus Selector : BusSelector  OutputSignals=velocity_RL,rotation_RL,inclination_RL
  Constant : Constant  Value=0
  MATLAB Function : MATLAB Function  TreatAsAtomicUnit=on
  Magic formula : MATLAB Function  TreatAsAtomicUnit=on
  Scope : Scope
  Scope1 : Scope
  Switch : Switch  Criteria=u2 > Threshold  Threshold=0.5  SaturateOnIntegerOverflow=off  InputSameDT=off
  norm : MATLAB Function  TreatAsAtomicUnit=on
  Force : Outport
  wires:
  Fz/1 -> Magic formula/1(Fz)
  Switch/1 -> Force/1
  norm/1(y) -> Switch/2
  Magic formula/1(Fy) -> Scope/1, Switch/1
  Constant/1 -> Switch/3
  Tyre data/1 -> Bus Selector/1
  MATLAB Function/1(theta) -> Magic formula/2(SA), Scope1/1  "Effective slip angle_RL"
  Bus Selector/1 -> [Speed], MATLAB Function/1(u)  "<velocity_RL>"
  [Speed] -> norm/1(u)
  Bus Selector/2 -> MATLAB Function/2(r)  "<rotation_RL>"
  Bus Selector/3 -> Magic formula/3(Camber)  "<inclination_RL>"

== system model2bf/Tyre_RL/Subsystem ==
  Constant{,1..3} (4 alike) : Constant  Value=0
  Vector Concatenate : Concatenate  NumInputs=3
  Vector Concatenate1 : Concatenate  NumInputs=3
  Vector Concatenate3 : Concatenate  NumInputs=3
  inclination_RL : Outport
  inclination_RL1 : Outport  Port=2
  inclination_RL2 : Outport  Port=3
  inclination_RL3 : Outport  Port=4
  wires:
  Constant/1 -> Vector Concatenate/3, Vector Concatenate/2, Vector Concatenate/1
  Vector Concatenate/1 -> inclination_RL/1  "inclination_RL"
  Constant1/1 -> Vector Concatenate1/3, Vector Concatenate1/2, Vector Concatenate1/1
  Vector Concatenate1/1 -> inclination_RL1/1  "inclination_RL"
  Constant2/1 -> inclination_RL2/1  "inclination_RL"
  Constant3/1 -> Vector Concatenate3/3, Vector Concatenate3/2, Vector Concatenate3/1
  Vector Concatenate3/1 -> inclination_RL3/1  "inclination_RL"

== system model2bf/Tyre_RR/Magic formula subsystem ==
  note: positive force = to the left
  Fz : Inport
  Tyre data : Inport  Port=2
  Bus Selector : BusSelector  OutputSignals=velocity_RR,rotation_RR,inclination_RR
  Constant : Constant  Value=0
  MATLAB Function : MATLAB Function  TreatAsAtomicUnit=on
  Magic formula : MATLAB Function  TreatAsAtomicUnit=on
  Scope : Scope
  Scope1 : Scope
  Switch : Switch  Criteria=u2 > Threshold  Threshold=0.5  SaturateOnIntegerOverflow=off  InputSameDT=off
  norm : MATLAB Function  TreatAsAtomicUnit=on
  Force : Outport
  wires:
  Fz/1 -> Magic formula/1(Fz)
  Switch/1 -> Force/1
  norm/1(y) -> Switch/2
  Magic formula/1(Fy) -> Scope/1, Switch/1
  Constant/1 -> Switch/3
  Tyre data/1 -> Bus Selector/1
  MATLAB Function/1(theta) -> Scope1/1, Magic formula/2(SA)  "Effective slip angle_RR"
  Bus Selector/1 -> [Speed], MATLAB Function/1(u)  "<velocity_RR>"
  [Speed] -> norm/1(u)
  Bus Selector/2 -> MATLAB Function/2(r)  "<rotation_RR>"
  Bus Selector/3 -> Magic formula/3(Camber)  "<inclination_RR>"

== system model2bf/Tyre_RR/Subsystem ==
  Constant{,1..3} (4 alike) : Constant  Value=0
  Vector Concatenate : Concatenate  NumInputs=3
  Vector Concatenate1 : Concatenate  NumInputs=3
  Vector Concatenate3 : Concatenate  NumInputs=3
  inclination_RL : Outport
  inclination_RL1 : Outport  Port=2
  inclination_RL2 : Outport  Port=3
  inclination_RL3 : Outport  Port=4
  wires:
  Constant/1 -> Vector Concatenate/3, Vector Concatenate/2, Vector Concatenate/1
  Vector Concatenate/1 -> inclination_RL/1  "inclination_RL"
  Constant1/1 -> Vector Concatenate1/3, Vector Concatenate1/2, Vector Concatenate1/1
  Vector Concatenate1/1 -> inclination_RL1/1  "inclination_RL"
  Constant2/1 -> inclination_RL2/1  "inclination_RL"
  Constant3/1 -> Vector Concatenate3/3, Vector Concatenate3/2, Vector Concatenate3/1
  Vector Concatenate3/1 -> inclination_RL3/1  "inclination_RL"

== system model2bf/Driveline/Subsystem3/Subsystem ==
  Regen_demand : Inport
  Regen_Limit : Inport  Port=2
  Constant : Constant  Value=0
  Saturation Dynamic : simulink/Discontinuities/Saturation Dynamic  OutMin=[]  OutMax=[]  OutDataTypeStr=Inherit: Same as second input  OutDataType=fixdt(1, 16)  OutScaling=2^-10  DoSatur=off
  Regen_Trq : Outport
  wires:
  Constant/1 -> Saturation Dynamic/1
  Regen_Limit/1 -> Saturation Dynamic/3
  Saturation Dynamic/1 -> Regen_Trq/1
  Regen_demand/1 -> Saturation Dynamic/2

== system model2bf/Driveline/Subsystem3/Torque limit ==
  Throttle (%) : Inport
  Motor torque (Nm) : Inport  Port=2
  Min : MinMax  Inputs=2
  Motor_Max_Trq : Constant  Value=motor.maxtorque
  Product : Product
  Scope : Scope
  Two driven wheels : Gain  Gain=-0.5
  Regen_trq_limit : Outport
  Trq_Dmd : Outport  Port=2
  wires:
  Motor_Max_Trq/1 -> Min/1
  Min/1 -> Two driven wheels/1, Product/2
  Throttle (%)/1 -> Product/1
  Two driven wheels/1 -> Regen_trq_limit/1
  Product/1 -> Trq_Dmd/1
  Motor torque (Nm)/1 -> Scope/1, Min/2

== matlab function model2bf/Tyre_RL/Magic formula subsystem/MATLAB Function ==
  data: u input; theta output; r input
function theta = fcn(u, r)
% function that calculates the slip angle of the tyre without considering
% the steering input given from the driver
% u = speed of the tyre [ux, uy, uz]
% r = rotation sequence of the tyre frame system [anglearound z-axis, anglearound x-axis, anglearound y-axis]

tyre_direction = exp(1i*r(1));
complexV = u(1) + u(2)*1j;
complexSlip = complexV/tyre_direction;
theta = angle(complexSlip);

== matlab function model2bf/Tyre_RL/Magic formula subsystem/Magic formula ==
  data: Fz input; SA input; Fy output; Camber input
function Fy = fcn(Fz, SA, Camber)
% Magic formula based on the data extracted from the TTC files

%valuesOfCamber = [0, 2, 4]
if abs(Camber) < 2
    params = [0.198719422442493, 1.649465431297653, 2.373300291953069, 0.233708623192915];
elseif 2 < abs(Camber) && abs(Camber)< 4
    params =[0.198225281942057, 1.660247836348132, 2.603573409360138, 0.381647688805729];
else
    params = [0.208412365438189, 1.632235951563173, 2.790064934147678, 0.398583330098178];
end
Fy = Fz * (params(3) * sin(params(2) * atan(params(1) * SA - params(4) * (params(1) * SA - atan(params(1) * SA)))));

== matlab function model2bf/Tyre_RL/Magic formula subsystem/norm ==
  data: u input; y output
function y = fcn(u)
y = norm(u);

== matlab function model2bf/Tyre_FL/Magic formula subsystem/MATLAB Function ==
  data: u input; theta output; r input
function theta = fcn(u, r)
% function that calculates the slip angle of the tyre without considering
% the steering input given from the driver
% u = speed of the tyre [ux, uy, uz]
% r = rotation sequence of the tyre frame system [anglearound z-axis, anglearound x-axis, anglearound y-axis]

tyre_direction = exp(1i*r(1));
complexV = u(1) + u(2)*1j;
complexSlip = complexV/tyre_direction;
theta = angle(complexSlip);

== matlab function model2bf/Steering function ==
  data: theta input; mean_angle output; right_angle output; left_angle output
 function [mean_angle, right_angle, left_angle] = steer(theta)

    % theta = steering wheel angle [-180, 180]°     positive : right turn !
    
    % mean_angle = mean steering angle [-30, 30]°
    % right_angle = right wheel steering angle
    % left_angle = left wheel steering angle

    b = 1;  % length of the front axle
    l = 3;  % distance between rear and front axles
    
    SR = 180/30;    % steering ratio 180°/30°

    mean_angle = theta/SR;

    right_angle = atand(1 /(cotd(mean_angle) + b/2/l));
    left_angle = atand(1 /(cotd(mean_angle) - b/2/l));
end

== matlab function model2bf/Tyre_FL/Magic formula subsystem/Magic formula ==
  data: Fz input; SA input; Fy output; Camber input
function Fy = fcn(Fz, SA, Camber)
% Magic formula based on the data extracted from the TTC files

%valuesOfCamber = [0, 2, 4]
if abs(Camber) < 2
    params = [0.198719422442493, 1.649465431297653, 2.373300291953069, 0.233708623192915];
elseif 2 < abs(Camber) && abs(Camber)< 4
    params =[0.198225281942057, 1.660247836348132, 2.603573409360138, 0.381647688805729];
else
    params = [0.208412365438189, 1.632235951563173, 2.790064934147678, 0.398583330098178];
end
Fy = Fz * (params(3) * sin(params(2) * atan(params(1) * SA - params(4) * (params(1) * SA - atan(params(1) * SA)))));

== matlab function model2bf/Tyre FR/Magic formula subsystem/MATLAB Function ==
  data: u input; theta output; r input
function theta = fcn(u, r)
% function that calculates the slip angle of the tyre without considering
% the steering input given from the driver
% u = speed of the tyre [ux, uy, uz]
% r = rotation sequence of the tyre frame system [anglearound z-axis, anglearound x-axis, anglearound y-axis]
tyre_direction = exp(1i*r(1));
complexV = u(1) + u(2)*1j;
complexSlip = complexV/tyre_direction;
theta = angle(complexSlip);
